simulink model "cannonball"  (Simulink 3.00)
settings: Solver=ode45  StartTime=0.0  StopTime=1.5  RelTol=1e-3
values from neighbouring files (symbols this model uses):
  g = 9.81    [cannonballpar.m]    (also in pendcartpar.m = 1; pendragpar.m)
  kappa = rho*S*Cd/2    (= 0.007618)    [cannonballpar.m]    (also in pendragpar.m = 0.0003809)
  m = 1    [cannonballpar.m]    (also in pendcartpar.m; pendragpar.m = 0.01)
libraries: simulink3 x1

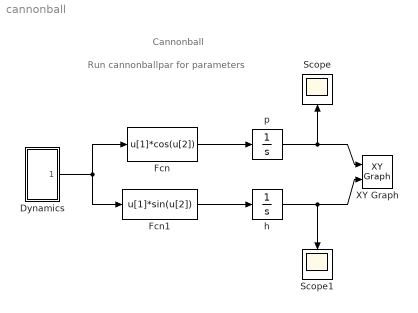
== system cannonball ==
  note: Cannonball
  note: Run cannonballpar for parameters
  Dynamics : Subsystem  Description=dynamics
  Fcn : Fcn  Expr=u[1]*cos(u[2])
  Fcn1 : Fcn  Expr=u[1]*sin(u[2])
  Scope : Scope
      settings: Orientation=up  TimeRange=auto  YMin=-5  YMax=5  SaveToWorkspace=off  SaveName=ScopeData
  Scope1 : Scope
      settings: Orientation=down  TimeRange=auto  YMin=-5  YMax=5  SaveToWorkspace=off  SaveName=ScopeData
  XY Graph : simulink3/Sinks/XY Graph  xmin=0  xmax=12  ymin=-2  ymax=4  st=-1
  h : Integrator  ExternalReset=none  InitialConditionSource=internal  InitialCondition=0  LimitOutput=off  UpperSaturationLimit=inf  LowerSaturationLimit=-inf  ShowSaturationPort=off  ShowStatePort=off  AbsoluteTolerance=auto
  p : Integrator  ExternalReset=none  InitialConditionSource=internal  InitialCondition=0  LimitOutput=off  UpperSaturationLimit=inf  LowerSaturationLimit=-inf  ShowSaturationPort=off  ShowStatePort=off  AbsoluteTolerance=auto
  wires:
  Fcn/1 -> p/1
  Fcn1/1 -> h/1
  p/1 -> XY Graph/1, Scope/1
  h/1 -> XY Graph/2, Scope1/1
  Dynamics/1(Out1) -> Fcn/1, Fcn1/1

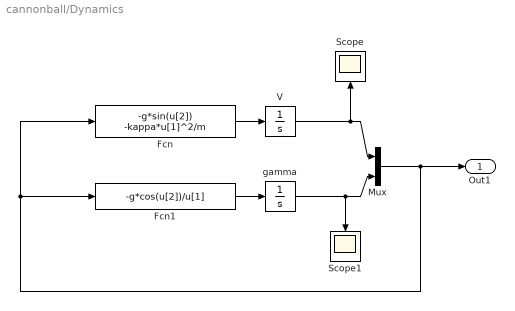
== system cannonball/Dynamics ==
  Fcn : Fcn  Expr=-g*sin(u[2]) -kappa*u[1]^2/m
  Fcn1 : Fcn  Expr=-g*cos(u[2])/u[1]
  Mux : Mux  Inputs=2
  Scope : Scope
      settings: Orientation=up  TimeRange=auto  YMin=-5  YMax=5  SaveToWorkspace=off  SaveName=ScopeData
  Scope1 : Scope
      settings: Orientation=down  TimeRange=auto  YMin=-5  YMax=5  SaveToWorkspace=off  SaveName=ScopeData
  V : Integrator  ExternalReset=none  InitialConditionSource=internal  InitialCondition=10  LimitOutput=off  UpperSaturationLimit=inf  LowerSaturationLimit=-inf  ShowSaturationPort=off  ShowStatePort=off  AbsoluteTolerance=auto
  gamma : Integrator  ExternalReset=none  InitialConditionSource=internal  InitialCondition=pi/4  LimitOutput=off  UpperSaturationLimit=inf  LowerSaturationLimit=-inf  ShowSaturationPort=off  ShowStatePort=off  AbsoluteTolerance=auto
  Out1 : Outport  Port=1
  wires:
  Fcn/1 -> V/1
  V/1 -> Mux/1, Scope/1
  Fcn1/1 -> gamma/1
  gamma/1 -> Mux/2, Scope1/1
  Mux/1 -> Out1/1, Fcn1/1, Fcn/1
